simulink model "foc_qep_sim"  (R2025b)
settings: Solver=FixedStepDiscrete  StartTime=0.0  StopTime=6  RelTol=1e-3
InitFcn:
  | foc_qep_data;
values from neighbouring files (symbols this model uses):
  PI_params = mcb.getPIControllerParameters(pmsm, inverter, PU_System, T_pwm, 5*Ts, Ts_speed)    [foc_qep_data.m]
  PU_System = mcb.getPUSystemParameters(pmsm, inverter)    [foc_qep_data.m]
  Ts_motor = T_pwm/2    (= 2.5e-05)    [foc_qep_data.m]
  Ts_simulink = T_pwm/2    (= 2.5e-05)    [foc_qep_data.m]
undefined symbols (not defined in the file or in its folder): inverter, pmsm, target
libraries: mcbplantlib x1, autolibpmsmexterior x1

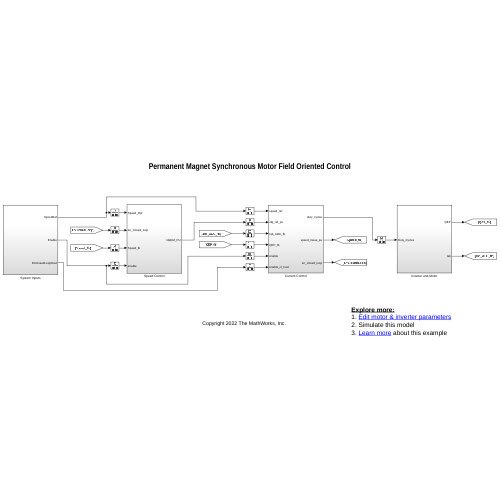
[thumbnail: Simulink's stored preview of the top-level diagram]
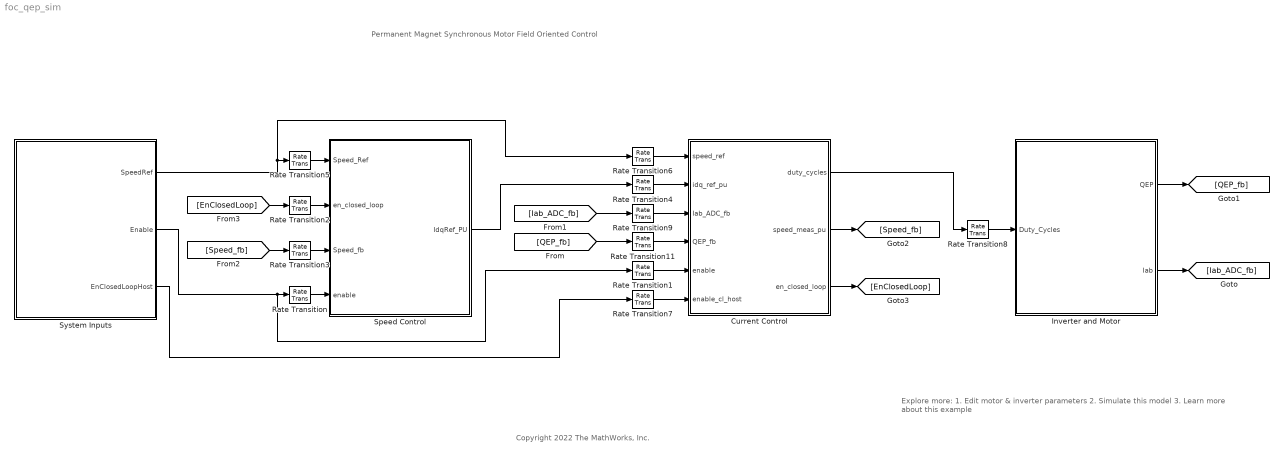
== system foc_qep_sim ==
  note: Permanent Magnet Synchronous Motor Field Oriented Control
  note: Copyright 2022 The MathWorks, Inc.
  note: Explore more:
      | 1. Edit motor & inverter parameters
      | 2. Simulate this model
      | 3. Learn more about this example
  Current Control : Subsystem
  Inverter and Motor : Subsystem
  Rate Transition{,2..3,5} (4 alike) : RateTransition  Deterministic=off  OutPortSampleTime=Ts_speed
  Rate Transition{1,4,6..7,9,11} (6 alike) : RateTransition  Deterministic=off  OutPortSampleTime=Ts
  Rate Transition8 : RateTransition  Deterministic=off
  Speed Control : Subsystem
  System Inputs : Subsystem
  wires:
  Rate Transition8/1 -> Inverter and Motor/1(Duty_Cycles)
  Rate Transition4/1 -> Current Control/2(idq_ref_pu)
  Rate Transition9/1 -> Current Control/3(Iab_ADC_fb)
  Rate Transition11/1 -> Current Control/4(QEP_fb)
  Rate Transition1/1 -> Current Control/5(enable)
  Rate Transition6/1 -> Current Control/1(speed_ref)
  Rate Transition7/1 -> Current Control/6(enable_cl_host)
  Current Control/1(duty_cycles) -> Rate Transition8/1
  Inverter and Motor/2(Iab) -> [Iab_ADC_fb]
  Inverter and Motor/1(QEP) -> [QEP_fb]
  [Iab_ADC_fb] -> Rate Transition9/1
  [QEP_fb] -> Rate Transition11/1
  Current Control/2(speed_meas_pu) -> [Speed_fb]
  Current Control/3(en_closed_loop) -> [EnClosedLoop]
  [Speed_fb] -> Rate Transition3/1
  [EnClosedLoop] -> Rate Transition2/1
  System Inputs/1(SpeedRef) -> Rate Transition5/1, Rate Transition6/1
  System Inputs/2(Enable) -> Rate Transition1/1, Rate Transition/1
  Rate Transition5/1 -> Speed Control/1(Speed_Ref)
  Rate Transition3/1 -> Speed Control/3(Speed_fb)
  Rate Transition/1 -> Speed Control/4(enable)
  Rate Transition2/1 -> Speed Control/2(en_closed_loop)
  Speed Control/1(IdqRef_PU) -> Rate Transition4/1
  System Inputs/3(EnClosedLoopHost) -> Rate Transition7/1

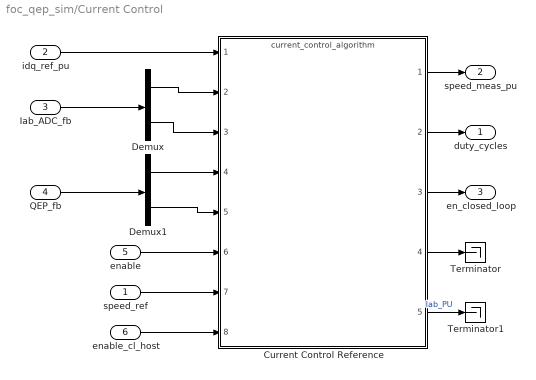
== system foc_qep_sim/Current Control ==
  speed_ref : Inport
  idq_ref_pu : Inport  Port=2
  Iab_ADC_fb : Inport  Port=3
  QEP_fb : Inport  Port=4
  enable : Inport  Port=5
  enable_cl_host : Inport  Port=6
  Current Control Reference : ModelReference  ModelNameDialog=current_control_algorithm  SimulationMode=Normal  ModelReferenceVersion=9.0
  Demux : Demux  Outputs=2
  Demux1 : Demux  Outputs=2
  Terminator : Terminator
  Terminator1 : Terminator
  duty_cycles : Outport
  speed_meas_pu : Outport  Port=2
  en_closed_loop : Outport  Port=3
  wires:
  Demux1/1 -> Current Control Reference/4
  QEP_fb/1 -> Demux1/1
  enable/1 -> Current Control Reference/6
  Demux/2 -> Current Control Reference/3
  Demux/1 -> Current Control Reference/2
  idq_ref_pu/1 -> Current Control Reference/1
  Iab_ADC_fb/1 -> Demux/1
  Current Control Reference/5 -> Terminator1/1  "Iab_PU"
  Current Control Reference/1 -> speed_meas_pu/1
  Current Control Reference/2 -> duty_cycles/1
  Current Control Reference/3 -> en_closed_loop/1
  Current Control Reference/4 -> Terminator/1
  enable_cl_host/1 -> Current Control Reference/8
  Demux1/2 -> Current Control Reference/5
  speed_ref/1 -> Current Control Reference/7

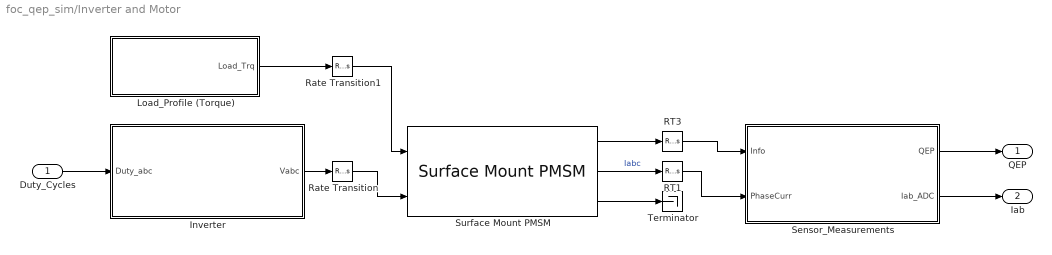
== system foc_qep_sim/Inverter and Motor ==
  Duty_Cycles : Inport
  Inverter : Subsystem
  Load_Profile (Torque) : Subsystem
  RT1 : RateTransition  Deterministic=off  OutPortSampleTime=Ts_simulink
  RT3 : RateTransition  Deterministic=off  OutPortSampleTime=Ts_simulink
  Rate Transition : RateTransition  Deterministic=off  OutPortSampleTime=Ts_motor
  Rate Transition1 : RateTransition  Deterministic=off  OutPortSampleTime=Ts_motor
  Sensor_Measurements : Subsystem
  Surface Mount PMSM : autolibpmsmexterior/Surface Mount PMSM  port_config=Torque  sim_type=Discrete  Ts=Ts_motor  P=pmsm.p  Rs=pmsm.Rs + inverter.R_board  Ldq_=pmsm.Ld  KConstText=Permanent flux linkage constant (lambda_pm):  lambda_pm=pmsm.FluxPM  Ke=159.9771  Kt=1.323  mechanical=[pmsm.J, pmsm.B, 0]  idq0=[0 0]  theta_init=0  omega_init=0  KConst=pmsm.FluxPM  lambda_pm_calc=pmsm.FluxPM  RefBlkName='autolibpmsmexterior/Surface Mount PMSM'  aMode=5  Ldq="[0.0002      0.0002]"
  Terminator : Terminator
  QEP : Outport  VectorParamsAs1DForOutWhenUnconnected=off
  Iab : Outport  Port=2  VectorParamsAs1DForOutWhenUnconnected=off
  wires:
  Sensor_Measurements/1(QEP) -> QEP/1
  Load_Profile (Torque)/1(Load_Trq) -> Rate Transition1/1
  Rate Transition1/1 -> Surface Mount PMSM/1
  Surface Mount PMSM/2 -> RT1/1  "Iabc"
  Duty_Cycles/1 -> Inverter/1(Duty_abc)
  Surface Mount PMSM/3 -> Terminator/1
  Inverter/1(Vabc) -> Rate Transition/1
  Rate Transition/1 -> Surface Mount PMSM/2
  RT3/1 -> Sensor_Measurements/1(Info)
  Surface Mount PMSM/1 -> RT3/1
  RT1/1 -> Sensor_Measurements/2(PhaseCurr)
  Sensor_Measurements/2(Iab_ADC) -> Iab/1

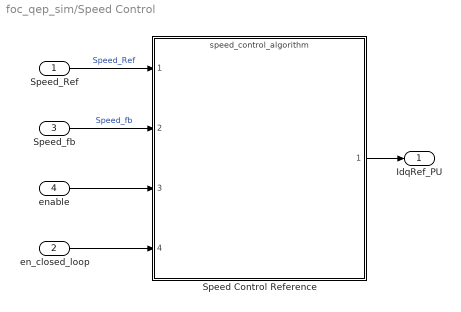
== system foc_qep_sim/Speed Control ==
  Speed_Ref : Inport
  en_closed_loop : Inport  Port=2
  Speed_fb : Inport  Port=3
  enable : Inport  Port=4
  Speed Control Reference : ModelReference  ModelNameDialog=speed_control_algorithm  SimulationMode=Normal  ModelReferenceVersion=9.0
  IdqRef_PU : Outport
  wires:
  Speed_fb/1 -> Speed Control Reference/2  "Speed_fb"
  en_closed_loop/1 -> Speed Control Reference/4
  Speed Control Reference/1 -> IdqRef_PU/1
  enable/1 -> Speed Control Reference/3
  Speed_Ref/1 -> Speed Control Reference/1  "Speed_Ref"

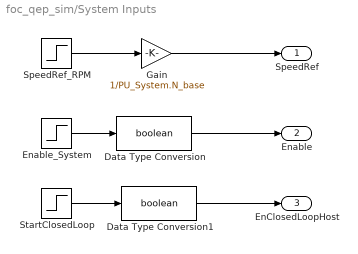
== system foc_qep_sim/System Inputs ==
  Data Type Conversion : DataTypeConversion  OutDataTypeStr=boolean  RndMeth=Simplest  SaturateOnIntegerOverflow=off
  Data Type Conversion1 : DataTypeConversion  OutDataTypeStr=boolean  RndMeth=Simplest  SaturateOnIntegerOverflow=off
  Enable_System : Step  Time=0  OutDataTypeStr=dataType  SampleTime=0.1
  Gain : Gain  Gain=1/PU_System.N_base  RndMeth=Simplest  OutDataTypeStr=Inherit: Same as input
  SpeedRef_RPM : Step  Time=2  Before=0.2*PU_System.N_base  After=0.5*PU_System.N_base  OutDataTypeStr=dataType  SampleTime=0.1
  StartClosedLoop : Step  Time=0  OutDataTypeStr=dataType  SampleTime=0.1
  SpeedRef : Outport
  Enable : Outport  Port=2
  EnClosedLoopHost : Outport  Port=3
  wires:
  Gain/1 -> SpeedRef/1
  SpeedRef_RPM/1 -> Gain/1
  Data Type Conversion1/1 -> EnClosedLoopHost/1
  Enable_System/1 -> Data Type Conversion/1
  Data Type Conversion/1 -> Enable/1
  StartClosedLoop/1 -> Data Type Conversion1/1

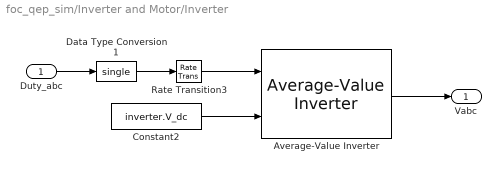
== system foc_qep_sim/Inverter and Motor/Inverter ==
  Duty_abc : Inport
  Average-Value Inverter : mcbplantlib/Average-Value Inverter
  Constant2 : Constant  Value=inverter.V_dc  OutDataTypeStr=single  SampleTime=-1
  Data Type Conversion1 : DataTypeConversion  OutDataTypeStr=single  RndMeth=Simplest  SaturateOnIntegerOverflow=off
  Rate Transition3 : RateTransition  Deterministic=off  OutPortSampleTime=Ts_inverter
  Vabc : Outport  VectorParamsAs1DForOutWhenUnconnected=off
  wires:
  Constant2/1 -> Average-Value Inverter/2
  Data Type Conversion1/1 -> Rate Transition3/1
  Duty_abc/1 -> Data Type Conversion1/1
  Rate Transition3/1 -> Average-Value Inverter/1
  Average-Value Inverter/1 -> Vabc/1

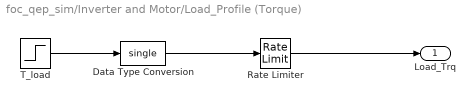
== system foc_qep_sim/Inverter and Motor/Load_Profile (Torque) ==
  Data Type Conversion : DataTypeConversion  OutDataTypeStr=single  SaturateOnIntegerOverflow=off  RndMeth=Floor
  Rate Limiter : RateLimiter  RisingSlewLimit=0.2  FallingSlewLimit=-0.2  SampleTimeMode=inherited
  T_load : Step  Time=4  Before=0.05*pmsm.T_rated  After=0.2*pmsm.T_rated  SampleTime=Ts_simulink
  Load_Trq : Outport  VectorParamsAs1DForOutWhenUnconnected=off
  wires:
  T_load/1 -> Data Type Conversion/1
  Data Type Conversion/1 -> Rate Limiter/1
  Rate Limiter/1 -> Load_Trq/1

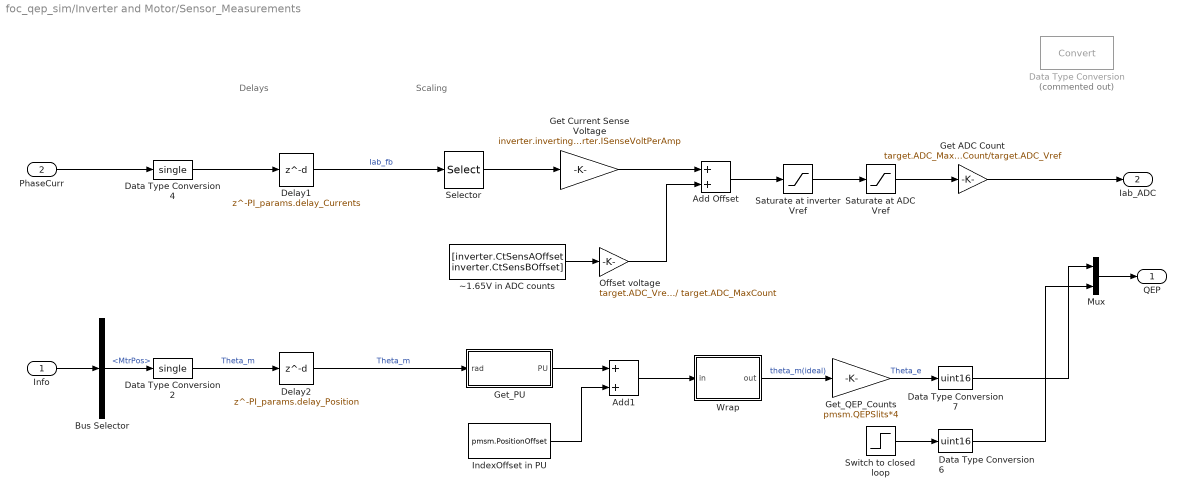
== system foc_qep_sim/Inverter and Motor/Sensor_Measurements ==
  note: Scaling
  note: Delays
  Info : Inport
  PhaseCurr : Inport  Port=2
  Add Offset : Sum  RndMeth=Simplest
  Add1 : Sum  RndMeth=Simplest
  Bus Selector : BusSelector  OutputSignals=MtrPos
  Data Type Conversion : DataTypeConversion  Commented=on  SaturateOnIntegerOverflow=off  RndMeth=Floor
  Data Type Conversion2 : DataTypeConversion  OutDataTypeStr=single  RndMeth=Simplest  SaturateOnIntegerOverflow=off
  Data Type Conversion4 : DataTypeConversion  OutDataTypeStr=single  RndMeth=Simplest  SaturateOnIntegerOverflow=off
  Data Type Conversion6 : DataTypeConversion  OutDataTypeStr=uint16  RndMeth=Simplest  SaturateOnIntegerOverflow=off
  Data Type Conversion7 : DataTypeConversion  OutDataTypeStr=uint16  RndMeth=Simplest  SaturateOnIntegerOverflow=off
  Delay1 : Delay  DelayLength=PI_params.delay_Currents
  Delay2 : Delay  DelayLength=PI_params.delay_Position
  Get ADC Count : Gain  Gain=target.ADC_MaxCount/target.ADC_Vref  OutMin=0  OutMax=target.ADC_MaxCount  OutDataTypeStr=Inherit: Inherit via back propagation  RndMeth=Simplest
  Get Current Sense Voltage : Gain  Gain=inverter.invertingAmp * inverter.ISenseVoltPerAmp  RndMeth=Simplest  OutDataTypeStr=Inherit: Same as input
  "Get_PU " : Subsystem
  Get_QEP_Counts : Gain  Gain=pmsm.QEPSlits*4  OutDataTypeStr=uint16  RndMeth=Simplest
  IndexOffset in PU : Constant  Value=pmsm.PositionOffset  OutDataTypeStr=single  SampleTime=-1
  Mux : Mux  Inputs=2
  Offset voltage : Gain  Gain=target.ADC_Vref / target.ADC_MaxCount  RndMeth=Simplest
  Saturate at ADC Vref : Saturate  UpperLimit=target.ADC_Vref  LowerLimit=0
  Saturate at inverter Vref : Saturate  UpperLimit=inverter.ISenseVref  LowerLimit=0
  Selector : Selector  InputPortWidth=3  IndexOptions=Index vector (dialog)  Indices=[1 2]  OutputSizes=1
  "Switch to closed loop " : Step  Time=0.1  SampleTime=Ts_motor
  Wrap : Subsystem
  ~1.65V in ADC counts : Constant  Value=[inverter.CtSensAOffset inverter.CtSensBOffset]  OutDataTypeStr=uint16  SampleTime=-1
  QEP : Outport  VectorParamsAs1DForOutWhenUnconnected=off
  Iab_ADC : Outport  Port=2  VectorParamsAs1DForOutWhenUnconnected=off
  wires:
  Delay1/1 -> Selector/1  "Iab_fb"
  Data Type Conversion4/1 -> Delay1/1
  PhaseCurr/1 -> Data Type Conversion4/1
  Info/1 -> Bus Selector/1
  Bus Selector/1 -> Data Type Conversion2/1  "<MtrPos>"
  Mux/1 -> QEP/1
  Data Type Conversion2/1 -> Delay2/1  "Theta_m"
  Add1/1 -> Wrap/1(in)
  Delay2/1 -> "Get_PU "/1(rad)  "Theta_m"
  Wrap/1(out) -> Get_QEP_Counts/1  "theta_m(ideal)"
  "Get_PU "/1(PU) -> Add1/1
  Get_QEP_Counts/1 -> Data Type Conversion7/1  "Theta_e"
  IndexOffset in PU/1 -> Add1/2
  "Switch to closed loop "/1 -> Data Type Conversion6/1
  Saturate at inverter Vref/1 -> Saturate at ADC Vref/1
  Saturate at ADC Vref/1 -> Get ADC Count/1
  Get Current Sense Voltage/1 -> Add Offset/1
  ~1.65V in ADC counts/1 -> Offset voltage/1
  Add Offset/1 -> Saturate at inverter Vref/1
  Offset voltage/1 -> Add Offset/2
  Selector/1 -> Get Current Sense Voltage/1
  Data Type Conversion7/1 -> Mux/1
  Data Type Conversion6/1 -> Mux/2
  Get ADC Count/1 -> Iab_ADC/1

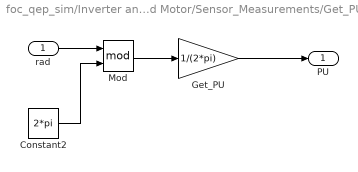
== system foc_qep_sim/Inverter and Motor/Sensor_Measurements/Get_PU  ==
  rad : Inport
  Constant2 : Constant  Value=2*pi  OutDataTypeStr=single  SampleTime=-1
  Get_PU : Gain  Gain=1/(2*pi)  RndMeth=Simplest  OutDataTypeStr=Inherit: Same as input
  Mod : Math  Operator=mod
  PU : Outport  VectorParamsAs1DForOutWhenUnconnected=off
  wires:
  rad/1 -> Mod/1
  Constant2/1 -> Mod/2
  Mod/1 -> Get_PU/1
  Get_PU/1 -> PU/1

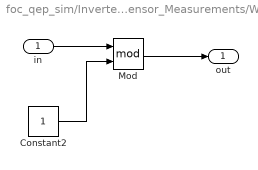
== system foc_qep_sim/Inverter and Motor/Sensor_Measurements/Wrap ==
  in : Inport
  Constant2 : Constant  OutDataTypeStr=single  SampleTime=-1
  Mod : Math  Operator=mod
  out : Outport  VectorParamsAs1DForOutWhenUnconnected=off
  wires:
  in/1 -> Mod/1
  Constant2/1 -> Mod/2
  Mod/1 -> out/1
